simulink model "mech_interface_crate_trans"  (R2015a)
settings: Solver=ode15s  StartTime=0.0  StopTime=10.0  RelTol=1e-3
PostLoadFcn:
  | mech_crate_transfer_param
model workspace (MAT data in the model file):
  A_a = 0.05
  A_b = 0.5
  A_c = 0.05
  M_a = 1
  I_a = [0.0841666666667  0  0; 0  0.00166666666667  0; 0  0  0.0841666666667]
  C_a = 0.25
  C_b = 0.05
  C_c = 0.05
  M_c = 5
  I_c = [0.00833333333333  0  0; 0  0.108333333333  0; 0  0  0.108333333333]
undefined symbols (not defined in the file): sigbuilder_block
libraries: mblibv1 x17, fl_lib x10, nesl_utility x4
Description:
  | Hydraulically Operated Crate Transfer Mechanism
  | 
  | This example shows a hydraulically operated four bar linkage that transfers crates between platforms of different heights. The Body Force Interface subsystem uses a Prismatic-Translational Interface block with Spherical and Prismatic joints to connect a hydraulic cylinder between Ground C and Body B.
  | 
  | The hydraulic circuit is modeled in Simscape(TM). The rest of the mechanism is modeled in SimMechanics(TM).
  | 
  | Copyright 2008-2014 The MathWorks, Inc.
settings Model: CovSFcnEnable=off  Creator=MathWorks  LastModifiedBy=psanghvi
settings SolverCC: MaxOrder=3  SolverResetMethod=Robust
settings DataIOCC: SignalLoggingSaveFormat=ModelDataLogs  OutputOption=SpecifiedOutputTimes  OutputTimes=[0:0.05:10]
settings OptimizationCC: ExpressionDepthLimit=2147483647  InitFltsAndDblsToZero=on
settings DebuggingCC: AlgebraicLoopMsg=none  UnderspecifiedInitializationDetection=Classic  MergeDetectMultiDrivingBlocksExec=none  FcnCallInpInsideContextMsg=UseLocalSettings  StateNameClashWarn=warning
settings GRTTargetCC: TargetFcnLib=ansi_tfl_tmw_new.mat  CombineOutputUpdateFcns=off  GRTInterface=on
settings SimMechanicsCC: WarnOnRedundantConstraints=off  VisOnUpdateDiagram=on  VisDuringSimulation=on  AnimationDelay=0  LastVizWinPosition=[680 677 559 420]  CamPosition=[0.138538;0.4511;12.0268;]  CamTarget=[0.138538;0.4511;0;]  CamUpVector=[0;1;0;]  CamHeight=1.87351  VisBackgroundColor=[0.9;0.9;0.95;]  DefaultBodyColor=[1;0;0;]  OVRRIDBodyVisualizationType=CONVHULL

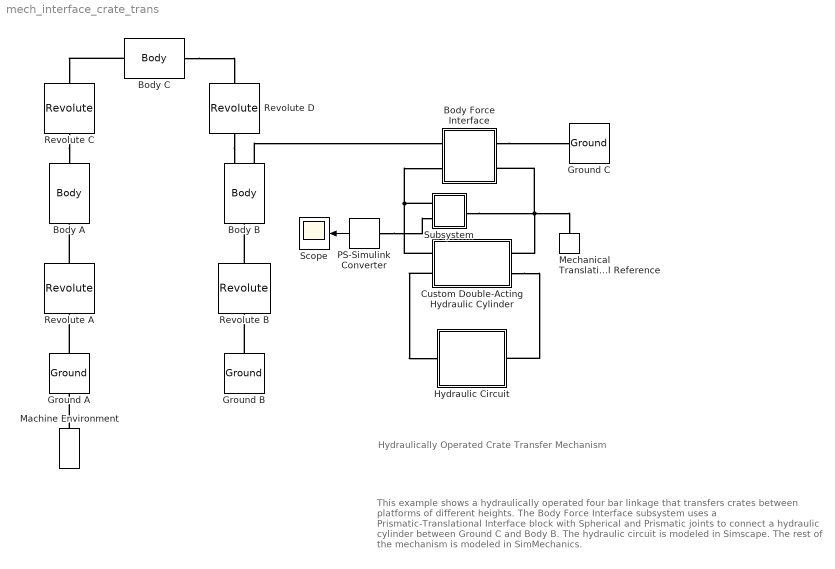
== system mech_interface_crate_trans ==
  note: Hydraulically Operated Crate Transfer Mechanism
  note: This example shows a hydraulically operated four bar linkage that
      | transfers crates between platforms of different heights. The Body Force Interface
      | subsystem uses a Prismatic-Translational Interface block with Spherical and Prismatic
      | joints to connect a hydraulic cylinder between Ground C and Body B.
      |
      | The hydraulic circuit is modeled in Simscape.
      | The rest of the mechanism is modeled in SimMechanics.
  Body A : mblibv1/Bodies/Body  LConnTagsString=CS1  RConnTagsString=CS2  UpdateFromCAD=off  DialogClass=MechanicalBodyBlock  Mass=M_a  MassUnits=kg  InertiaUnits=kg*m^2  Inertia=I_a  Shape=Cylinder  ShapeDims=[1 1]  ShapeUnits=m  ShapeUse=false  Density=1  DensityUnits=kg/m^3  DensityUse=false  GraphicsMode=MACHINE_DEFAULT  BodyColorSelMode=MACHINE_DEFAULT  BodyColor=[1 0 0]  AttachedToCS=CG  CG=Left$CG$[0 A_b 0]$CS1$CS1$m$[0 0 0]$Euler X-Y-Z$deg$WORLD$false  WorkingFrames=Left$CS1$[0.0 0 0]$Adjoining$Adjoining$m$[0 0 0]$Euler X-Y-Z$deg$WORLD$true#Right$CS2$[0 2*A_b 0]$CS1$CS1$m$[0 0 0]$Euler X-Y-Z$deg$WORLD$true  CGPos=[0 A_b 0]  CGRot=[0 0 0]  CS0Pos=[]  CS0Rot=[]  CS1Pos=[0.0 0 0]  CS1Rot=[0 0 0]  CS2Pos=[0 2*A_b 0]  CS2Rot=[0 0 0]  CS3Pos=[]  CS3Rot=[]  CS4Pos=[]  CS4Rot=[]  CS5Pos=[]  CS5Rot=[]  CS6Pos=[]  CS6Rot=[]  CS7Pos=[]  CS7Rot=[]  CS8Pos=[]  CS8Rot=[]  CS9Pos=[]  CS9Rot=[]  CS10Pos=[]  CS10Rot=[]  CS11Pos=[]  CS11Rot=[]  CS12Pos=[]  CS12Rot=[]  CS13Pos=[]  CS13Rot=[]  CS14Pos=[]  CS14Rot=[]  CS15Pos=[]  CS15Rot=[]  CS16Pos=[]  CS16Rot=[]  CS17Pos=[]  CS17Rot=[]  CS18Pos=[]  CS18Rot=[]  CS19Pos=[]  CS19Rot=[]  CS20Pos=[]  CS20Rot=[]
  Body B : mblibv1/Bodies/Body  LConnTagsString=CS1  RConnTagsString=CS2|CS3  UpdateFromCAD=off  DialogClass=MechanicalBodyBlock  Mass=M_a  MassUnits=kg  InertiaUnits=kg*m^2  Inertia=I_a  Shape=Cylinder  ShapeDims=[1 1]  ShapeUnits=m  ShapeUse=false  Density=1  DensityUnits=kg/m^3  DensityUse=false  GraphicsMode=MACHINE_DEFAULT  BodyColorSelMode=MACHINE_DEFAULT  BodyColor=[1 0 0]  AttachedToCS=CG  CG=Left$CG$[0 A_b 0]$CS1$CS1$m$[0 0 0]$Euler X-Y-Z$deg$WORLD$false  WorkingFrames=Left$CS1$[0 0 0]$Adjoining$Adjoining$m$[0 0 0]$Euler X-Y-Z$deg$WORLD$true#Right$CS2$[0 2*A_b 0]$CS1$CS1$m$[0 0 0]$Euler X-Y-Z$deg$WORLD$true#Right$CS3$[0 0 0]$CG$CG$m$[0 0 0]$Euler X-Y-Z$deg$WORLD$true  CGPos=[0 A_b 0]  CGRot=[0 0 0]  CS0Pos=[]  CS0Rot=[]  CS1Pos=[0 0 0]  CS1Rot=[0 0 0]  CS2Pos=[0 2*A_b 0]  CS2Rot=[0 0 0]  CS3Pos=[0 0 0]  CS3Rot=[0 0 0]  CS4Pos=[]  CS4Rot=[]  CS5Pos=[]  CS5Rot=[]  CS6Pos=[]  CS6Rot=[]  CS7Pos=[]  CS7Rot=[]  CS8Pos=[]  CS8Rot=[]  CS9Pos=[]  CS9Rot=[]  CS10Pos=[]  CS10Rot=[]  CS11Pos=[]  CS11Rot=[]  CS12Pos=[]  CS12Rot=[]  CS13Pos=[]  CS13Rot=[]  CS14Pos=[]  CS14Rot=[]  CS15Pos=[]  CS15Rot=[]  CS16Pos=[]  CS16Rot=[]  CS17Pos=[]  CS17Rot=[]  CS18Pos=[]  CS18Rot=[]  CS19Pos=[]  CS19Rot=[]  CS20Pos=[]  CS20Rot=[]
  Body C : mblibv1/Bodies/Body  LConnTagsString=CS1  RConnTagsString=CS2  UpdateFromCAD=off  DialogClass=MechanicalBodyBlock  Mass=M_c  MassUnits=kg  InertiaUnits=kg*m^2  Inertia=I_c  Shape=Cylinder  ShapeDims=[1 1]  ShapeUnits=m  ShapeUse=false  Density=1  DensityUnits=kg/m^3  DensityUse=false  GraphicsMode=MACHINE_DEFAULT  BodyColorSelMode=MACHINE_DEFAULT  BodyColor=[1 0 0]  AttachedToCS=CG  CG=Left$CG$[C_a 0 0]$CS1$CS1$m$[0 0 0]$Euler X-Y-Z$deg$WORLD$false  WorkingFrames=Left$CS1$[0.0 0 0]$Adjoining$Adjoining$m$[0 0 0]$Euler X-Y-Z$deg$WORLD$true#Right$CS2$[2*C_a 0 0]$CS1$CS1$m$[0 0 0]$Euler X-Y-Z$deg$WORLD$true  CGPos=[C_a 0 0]  CGRot=[0 0 0]  CS0Pos=[]  CS0Rot=[]  CS1Pos=[0.0 0 0]  CS1Rot=[0 0 0]  CS2Pos=[2*C_a 0 0]  CS2Rot=[0 0 0]  CS3Pos=[]  CS3Rot=[]  CS4Pos=[]  CS4Rot=[]  CS5Pos=[]  CS5Rot=[]  CS6Pos=[]  CS6Rot=[]  CS7Pos=[]  CS7Rot=[]  CS8Pos=[]  CS8Rot=[]  CS9Pos=[]  CS9Rot=[]  CS10Pos=[]  CS10Rot=[]  CS11Pos=[]  CS11Rot=[]  CS12Pos=[]  CS12Rot=[]  CS13Pos=[]  CS13Rot=[]  CS14Pos=[]  CS14Rot=[]  CS15Pos=[]  CS15Rot=[]  CS16Pos=[]  CS16Rot=[]  CS17Pos=[]  CS17Rot=[]  CS18Pos=[]  CS18Rot=[]  CS19Pos=[]  CS19Rot=[]  CS20Pos=[]  CS20Rot=[]
  Body Force Interface : Subsystem
  Custom Double-Acting Hydraulic Cylinder : Subsystem  mask(Hydraulic Double-Acting Cylinder, Custom Model){area_A=0.001, area_B=5e-4, stroke=1, init_pos=0.5, stiffness=1e6, damping=150}
      mask prompts: area_A "Area A (m^2)"; area_B "Area B (m^2)"; stroke "Stroke (m)"; init_pos "Initial position (m)"; stiffness "Contact stiffness (N/m)"; damping "Contact damping (N*s/m)"
      mask help: The model is built entirely of Foundation Library blocks and accounts for hard stops and fluid consumption due to piston motion.
      mask Display:
      | plot([127.790967235342;156.136468285695;156.136468285695;127.790967235342;127.790967235342], [113.618216710165;113.618216710165;56.927214609459;56.927214609459;113.618216710165])
      | plot([227.000220911577;227.000220911577;56.927214609459;56.927214609459;227.000220911577;227.000220911577], [99.4454661849886;113.618216710165;113.618216710165;56.927214609459;56.927214609459;71.0999651346356])
      | plot([156.136468285695;297.86397353746;297.86397353746;156.136468285695;156.136468285695], [99.4454661849886;99.4454661849886;71.0999651346356;71.0999651346356;99.4454661849886])
      | plot([56.927214609459;28.581713559106;56.927214609459], [113.618216710165;85.2727156598121;56.927214609459])
      | plot([28.581713559106;0.236212508752942], [85.2727156598121;85.2727156598121])
      | plot([297.86397353746;326.209474587813], [85.2727156598121;85.2727156598121])
      | plot([0.236212508752942;71.0999651346356;71.0999651346356], [28.581713559106;28.581713559106;56.927214609459])
      | plot([212.827470386401;212.827470386401;323.374924482778], [56.927214609459;28.581713559106;28.581713559106])
      | patch([0;326.445687096566;326.445687096566;0;0;0.472425017505884;0.472425017505884;325.97326207906;325.97326207906;0.472425017505884;0], [113.854429218918;113.854429218918;0;0;113.854429218918;113.382004201412;0.472425017505884;0.472425017505884;113.382004201412;113.382004201412;113.854429218918], [1;1;1])
      | ;
  Ground A : mblibv1/Bodies/Ground  UpdateFromCAD=off  LeftPortType=env  RightPortType=workingframe  PhysicalDomain=Mechanical  DialogClass=GroundBlock  CoordPosition=[0 0 0]  CoordPositionUnits=m  StateVectorMgrId=-1  MachineId=[0 0]  ShowEnvPort=on  ParameterChecksum=[2928839484, 1749172837, 1649258051, 964539551]  TopologyChecksum=[4150982369, 548530894, 407794712, 2107293366]
  Ground B : mblibv1/Bodies/Ground  UpdateFromCAD=off  LeftPortType=env  RightPortType=workingframe  PhysicalDomain=Mechanical  DialogClass=GroundBlock  CoordPosition=[0.5 0 0]  CoordPositionUnits=m  StateVectorMgrId=-1  MachineId=[0 0]  ShowEnvPort=off  ParameterChecksum=[0 0 0 0]  TopologyChecksum=[0 0 0 0]
  Ground C : mblibv1/Bodies/Ground  UpdateFromCAD=off  LeftPortType=env  RightPortType=workingframe  PhysicalDomain=Mechanical  DialogClass=GroundBlock  CoordPosition=[1 1 0]  CoordPositionUnits=m  StateVectorMgrId=-1  MachineId=[0 0]  ShowEnvPort=off  ParameterChecksum=[0 0 0 0]  TopologyChecksum=[0 0 0 0]
  Hydraulic Circuit : Subsystem
  Machine Environment : mblibv1/Bodies/Machine Environment  Tag=Factory ground  PortType=env  PhysicalDomain=Mechanical  DialogTemplateClass=MECH.MachineEnvironment  SyncWhenCopied=off  Gravity=[0 0 0]  GravityUnits=m/s^2  GravityAsSignal=off  Dimensionality=Auto-detect  AnalysisType=Forward dynamics  LinearAssemblyTolerance=1e-3  LinearAssemblyToleranceUnits=m  AngularAssemblyTolerance=1e-3  AngularAssemblyToleranceUnits=rad  ConstraintSolverType=Stabilizing  ConstraintRelTolerance=1e-4  ConstraintAbsTolerance=1e-4  UseRobustSingularityHandling=off  RedundancyAnalysisToleranceType=Automatically select tolerance  RedundancyAnalysisTolerance=1e-14  StatePerturbationType=Fixed  PerturbationSize=1e-5  VisualizeMachine=on  BodyVisualizationType=Use model default body geometries  BodyColorSelMode=Use model default  DefaultBodyColor=[1 0 0]
  Mechanical Translational Reference : fl_lib/Mechanical/Translational Elements/Mechanical Translational Reference
  PS-Simulink Converter : nesl_utility/PS-Simulink Converter  PhysicalDomain=network_engine_domain  SubClassName=ps_output  LeftPortType=input  RightPortType=output  PseudoPeriodic=off  Frequencies=[]  Unit=1  AffineConversion=off
  Revolute A : mblibv1/Joints/Revolute  LConnTagsString=__newl0  RConnTagsString=__newr0  UpdateFromCAD=off  NumSAPorts=0  CutJoint=off  MarkAsCut=off  Primitives=prismatic  PrimitiveProps=R1$World$[0 0 1]$revolute  DialogClass=JointBlock  R1Axis=[0 0 1]
  Revolute B : mblibv1/Joints/Revolute  LConnTagsString=__newl0  RConnTagsString=__newr0  UpdateFromCAD=off  NumSAPorts=0  CutJoint=off  MarkAsCut=off  Primitives=prismatic  PrimitiveProps=R1$World$[0 0 1]$revolute  DialogClass=JointBlock  R1Axis=[0 0 1]
  Revolute C : mblibv1/Joints/Revolute  LConnTagsString=__newl0  RConnTagsString=__newr0  UpdateFromCAD=off  NumSAPorts=0  CutJoint=off  MarkAsCut=off  Primitives=prismatic  PrimitiveProps=R1$WORLD$[0 0 1]$revolute  DialogClass=JointBlock  R1Axis=[0 0 1]
  Revolute D : mblibv1/Joints/Revolute  LConnTagsString=__newl0  RConnTagsString=__newr0  UpdateFromCAD=off  NumSAPorts=0  CutJoint=off  MarkAsCut=off  Primitives=prismatic  PrimitiveProps=R1$World$[0 0 1]$revolute  DialogClass=JointBlock  R1Axis=[0 0 1]
  Scope : Scope
      settings: TimeRange=10  YMin=-0.05  YMax=0.15
  Subsystem : Subsystem
  wires:
  PS-Simulink Converter/1 -> Scope/1
  connections:
  Ground A/RConn1 -- Revolute A/LConn1
  Revolute A/RConn1 -- Body A/LConn1
  Revolute B/RConn1 -- Body B/LConn1
  Ground B/RConn1 -- Revolute B/LConn1
  Revolute C/LConn1 -- Body A/RConn1
  Body C/LConn1 -- Revolute C/RConn1
  Revolute D/LConn1 -- Body B/RConn1
  Body C/RConn1 -- Revolute D/RConn1
  Body B/RConn2 -- Body Force Interface/LConn1
  Machine Environment/RConn1 -- Ground A/LConn1
  Custom Double-Acting Hydraulic Cylinder/RConn2 -- Hydraulic Circuit/LConn1
  Custom Double-Acting Hydraulic Cylinder/LConn2 -- Hydraulic Circuit/RConn1
  Custom Double-Acting Hydraulic Cylinder/LConn1 -- Body Force Interface/RConn2 -- Subsystem/RConn1 -- Mechanical Translational Reference/LConn1
  Custom Double-Acting Hydraulic Cylinder/RConn1 -- Subsystem/LConn1 -- Body Force Interface/LConn2
  Body Force Interface/RConn1 -- Ground C/RConn1
  PS-Simulink Converter/LConn1 -- Subsystem/LConn2

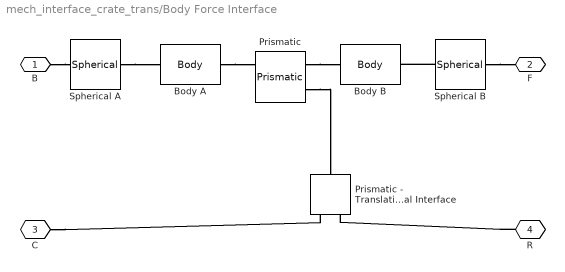
== system mech_interface_crate_trans/Body Force Interface ==
  Body A : mblibv1/Bodies/Body  LConnTagsString=CS1  RConnTagsString=CS2  UpdateFromCAD=off  DialogClass=MechanicalBodyBlock  Mass=0.1  MassUnits=kg  InertiaUnits=kg*m^2  Inertia=1e-3*[0.1 0 0;0 3 0; 0 0 3]  Shape=Cylinder  ShapeDims=[1 1]  ShapeUnits=m  ShapeUse=false  Density=1  DensityUnits=kg/m^3  DensityUse=false  GraphicsMode=MACHINE_DEFAULT  BodyColorSelMode=MACHINE_DEFAULT  BodyColor=[1 0 0]  AttachedToCS=CG  CG=Left$CG$[sqrt(2)*0.5/2 0 0]$CS1$CS1$m$[0 0 0]$Euler X-Y-Z$deg$CS1$false$none  WorkingFrames=Left$CS1$[0 0 0]$Adjoining$Adjoining$m$[0 0 45]$Euler X-Y-Z$deg$WORLD$true$none#Right$CS2$[sqrt(2)*0.5 0 0]$CS1$CS1$m$[0 0 0]$Euler X-Y-Z$deg$CS1$true$none  CGPos=[sqrt(2)*0.5/2 0 0]  CGRot=[0 0 0]  CS0Pos=[]  CS0Rot=[]  CS1Pos=[0 0 0]  CS1Rot=[0 0 45]  CS2Pos=[sqrt(2)*0.5 0 0]  CS2Rot=[0 0 0]  CS3Pos=[]  CS3Rot=[]  CS4Pos=[]  CS4Rot=[]  CS5Pos=[]  CS5Rot=[]  CS6Pos=[]  CS6Rot=[]  CS7Pos=[]  CS7Rot=[]  CS8Pos=[]  CS8Rot=[]  CS9Pos=[]  CS9Rot=[]  CS10Pos=[]  CS10Rot=[]  CS11Pos=[]  CS11Rot=[]  CS12Pos=[]  CS12Rot=[]  CS13Pos=[]  CS13Rot=[]  CS14Pos=[]  CS14Rot=[]  CS15Pos=[]  CS15Rot=[]  CS16Pos=[]  CS16Rot=[]  CS17Pos=[]  CS17Rot=[]  CS18Pos=[]  CS18Rot=[]  CS19Pos=[]  CS19Rot=[]  CS20Pos=[]  CS20Rot=[]
  Body B : mblibv1/Bodies/Body  LConnTagsString=CS1  RConnTagsString=CS2  UpdateFromCAD=off  DialogClass=MechanicalBodyBlock  Mass=0.1  MassUnits=kg  InertiaUnits=kg*m^2  Inertia=1e-3*[0.1 0 0;0 3 0; 0 0 3]  Shape=Cylinder  ShapeDims=[1 1]  ShapeUnits=m  ShapeUse=false  Density=1  DensityUnits=kg/m^3  DensityUse=false  GraphicsMode=MACHINE_DEFAULT  BodyColorSelMode=MACHINE_DEFAULT  BodyColor=[1 0 0]  AttachedToCS=CG  CG=Left$CG$[sqrt(2)*0.5/2 0 0]$CS1$CS1$m$[0 0 0]$Euler X-Y-Z$deg$CS1$false$none  WorkingFrames=Left$CS1$[-sqrt(2)*0.5 0 0]$Adjoining$Adjoining$m$[0 0 0]$Euler X-Y-Z$deg$Adjoining$true$none#Right$CS2$[sqrt(2)*0.5 0 0]$CS1$CS1$m$[0 0 0]$Euler X-Y-Z$deg$CS1$true$none  CGPos=[sqrt(2)*0.5/2 0 0]  CGRot=[0 0 0]  CS0Pos=[]  CS0Rot=[]  CS1Pos=[-sqrt(2)*0.5 0 0]  CS1Rot=[0 0 0]  CS2Pos=[sqrt(2)*0.5 0 0]  CS2Rot=[0 0 0]  CS3Pos=[]  CS3Rot=[]  CS4Pos=[]  CS4Rot=[]  CS5Pos=[]  CS5Rot=[]  CS6Pos=[]  CS6Rot=[]  CS7Pos=[]  CS7Rot=[]  CS8Pos=[]  CS8Rot=[]  CS9Pos=[]  CS9Rot=[]  CS10Pos=[]  CS10Rot=[]  CS11Pos=[]  CS11Rot=[]  CS12Pos=[]  CS12Rot=[]  CS13Pos=[]  CS13Rot=[]  CS14Pos=[]  CS14Rot=[]  CS15Pos=[]  CS15Rot=[]  CS16Pos=[]  CS16Rot=[]  CS17Pos=[]  CS17Rot=[]  CS18Pos=[]  CS18Rot=[]  CS19Pos=[]  CS19Rot=[]  CS20Pos=[]  CS20Rot=[]
  Prismatic : mblibv1/Joints/Prismatic  LConnTagsString=__newl0|SA1  RConnTagsString=__newr0|SA1  UpdateFromCAD=off  NumSAPorts=2  CutJoint=off  MarkAsCut=off  Primitives=prismatic  PrimitiveProps=P1$Base$[1 0 0]$prismatic  DialogClass=JointBlock  P1Axis=[1 0 0]
  Prismatic - Translational Interface : mblibv1/Interface  Elements/Prismatic - Translational Interface  UpdateFromCAD=off  DialogClass=PrismaticTranslationalInterface  Primitive=P1  InputFiltering=off  SimscapeFilterOrder=1  InputFilterTimeConstant=0.001
  "Spherical A " : mblibv1/Joints/Spherical  LConnTagsString=__newl0  RConnTagsString=__newr0  UpdateFromCAD=off  NumSAPorts=0  CutJoint=off  MarkAsCut=off  Primitives=spherical  PrimitiveProps=S$WORLD$[0 0 0]$spherical  DialogClass=JointBlock  SAxis=[0 0 0]
  Spherical B : mblibv1/Joints/Spherical  LConnTagsString=__newl0  RConnTagsString=__newr0  UpdateFromCAD=off  NumSAPorts=0  CutJoint=off  MarkAsCut=off  Primitives=spherical  PrimitiveProps=S$World$[0 0 0]$spherical  DialogClass=JointBlock  SAxis=[0 0 0]
  B : PMIOPort  Port=1  Side=Left
  F : PMIOPort  Port=2  Side=Right
  C : PMIOPort  Port=3  Side=Left
  R : PMIOPort  Port=4  Side=Right
  connections:
  R/RConn1 -- Prismatic - Translational Interface/LConn2
  C/RConn1 -- Prismatic - Translational Interface/LConn1
  B/RConn1 -- "Spherical A "/LConn1
  "Spherical A "/RConn1 -- Body A/LConn1
  Body A/RConn1 -- Prismatic/RConn1
  Prismatic/LConn1 -- Body B/LConn1
  Prismatic/LConn2 -- Prismatic - Translational Interface/RConn1
  Spherical B/RConn1 -- F/RConn1
  Spherical B/LConn1 -- Body B/RConn1

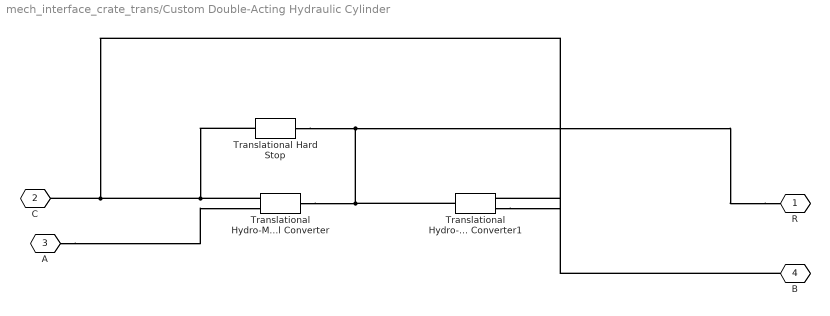
== system mech_interface_crate_trans/Custom Double-Acting Hydraulic Cylinder ==
  Translational Hydro-Mechanical Converter : fl_lib/Hydraulic/Hydraulic Elements/Translational Hydro-Mechanical Converter  area=area_A m^2  or=1  compressibility=0  init_pos=0 m  V_dead=1e-4 m^3  k_sh=1.4  initial_pressure=0 Pa
  Translational Hydro-Mechanical Converter1 : fl_lib/Hydraulic/Hydraulic Elements/Translational Hydro-Mechanical Converter  area=area_B m^2  or=2  compressibility=0  init_pos=0 m  V_dead=1e-4 m^3  k_sh=1.4  initial_pressure=0 Pa
  Translational Hard Stop : fl_lib/Mechanical/Translational Elements/Translational Hard Stop  upper_bnd=stroke - init_pos m  lower_bnd=-init_pos m  stiff_up=stiffness N/m  stiff_low=stiffness N/m  D_up=damping N/(m/s)  D_low=damping N/(m/s)  v_specify=off  v_priority=High  v=0 m/s  f_specify=off  f_priority=High  f=0 N  x_specify=on  x_priority=High  x=0 m
  R : PMIOPort  Tag=PMCPort  Port=1  Side=Right
  C : PMIOPort  Tag=PMCPort  Port=2  Side=Left
  A : PMIOPort  Tag=PMCPort  Port=3  Side=Left
  B : PMIOPort  Tag=PMCPort  Port=4  Side=Right
  connections:
  R/RConn1 -- Translational Hydro-Mechanical Converter1/RConn1 -- Translational Hydro-Mechanical Converter/RConn1 -- Translational Hard Stop/LConn1
  Translational Hydro-Mechanical Converter1/LConn1 -- Translational Hard Stop/RConn1 -- Translational Hydro-Mechanical Converter/LConn1 -- C/RConn1
  A/RConn1 -- Translational Hydro-Mechanical Converter/LConn2
  B/RConn1 -- Translational Hydro-Mechanical Converter1/LConn2

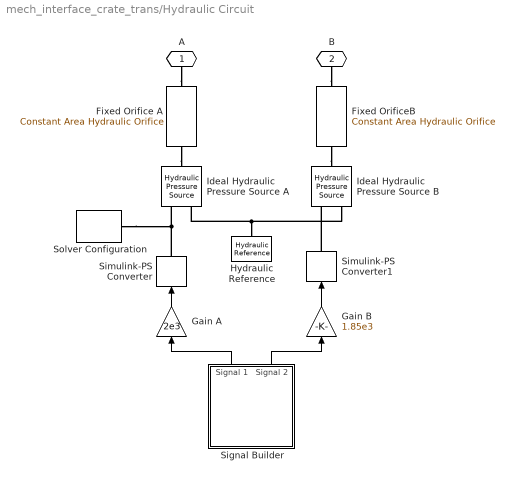
== system mech_interface_crate_trans/Hydraulic Circuit ==
  Fixed Orifice A : fl_lib/Hydraulic/Hydraulic Elements/Constant Area Hydraulic Orifice  area=1e-04 m^2  C_d=0.7  Re_cr=12  D_h=0.0113 m  p_cr=1 Pa  q_specify=off  q_priority=High  q=1 m^3/s  p_specify=off  p_priority=High  p=0 Pa
  Fixed OrificeB : fl_lib/Hydraulic/Hydraulic Elements/Constant Area Hydraulic Orifice  area=1e-04 m^2  C_d=0.7  Re_cr=12  D_h=0.0113 m  p_cr=1 Pa  q_specify=off  q_priority=High  q=1 m^3/s  p_specify=off  p_priority=High  p=0 Pa
  Gain A : Gain  Gain=2e3
  Gain B : Gain  Gain=1.85e3
  Hydraulic Reference : fl_lib/Hydraulic/Hydraulic Elements/Hydraulic Reference
  Ideal Hydraulic Pressure Source A : fl_lib/Hydraulic/Hydraulic Sources/Hydraulic Pressure Source
  Ideal Hydraulic Pressure Source B : fl_lib/Hydraulic/Hydraulic Sources/Hydraulic Pressure Source
  Signal Builder : Subsystem  Tag=STV Subsys  LoadFcn=sigbuilder_block('load');  StartFcn=sigbuilder_block('start');  StopFcn=sigbuilder_block('stop');  ClipboardFcn=sigbuilder_block('clipboard');  mask(Sigbuilder block){}
      mask help: Sigbuilder GUI
      mask init:
      | if ~strcmp(get_param(bdroot(gcbh),'SimulationStatus'),'stopped') tuvar = sigbuilder_block('maskInit'); end
      settings: CopyFcn=sigbuilder_block('copy');  DeleteFcn=sigbuilder_block('delete');  ModelCloseFcn=sigbuilder_block('modelClose');  PreSaveFcn=sigbuilder_block('preSave');  PauseFcn=sigbuilder_block('pause')  ContinueFcn=sigbuilder_block('continue')  NameChangeFcn=sigbuilder_block('namechange');  OpenFcn=sigbuilder_block('open',[388.5 359.25 550.5 371.25 ]);  CloseFcn=sigbuilder_block('close');
      mask Display: plot(0,0,100,100,[10,10,40,40,10],[80,20,20,80,80],[40,10],[50,50], [40,27,10],[65,72,56],[40,25,25,10],[28,28,43,43]);
  Simulink-PS Converter : nesl_utility/Simulink-PS Converter  PhysicalDomain=network_engine_domain  SubClassName=ps_input  LeftPortType=input  RightPortType=output  PseudoPeriodic=off  Frequencies=[]  NoiseDistribution=none  NoiseParameters=[]  Unit=N/m^2  AffineConversion=off  InputFiltering=off  SimscapeFilterOrder=1  InputFilterTimeConstant=.001  UdotUserProvided=0
  Simulink-PS Converter1 : nesl_utility/Simulink-PS Converter  PhysicalDomain=network_engine_domain  SubClassName=ps_input  LeftPortType=input  RightPortType=output  PseudoPeriodic=off  Frequencies=[]  NoiseDistribution=none  NoiseParameters=[]  Unit=N/m^2  AffineConversion=off  InputFiltering=off  SimscapeFilterOrder=1  InputFilterTimeConstant=.001  UdotUserProvided=0
  Solver Configuration : nesl_utility/Solver Configuration  PhysicalDomain=network_engine_domain  SubClassName=solver  LeftPortType=input  RightPortType=generic  Accelerate=off  Tones=[]  Harmonics=[]  SimulateNoise=off  Profile=off  UseLocalSampling=off  EnableSwitchedLinearOptims=on  FrequencyDomain=off  UseCCode=off  RelTol=0.001  AbsTol=1e-06  MinStep=1e-09  ToWorkspace=off  RevertToSquareIcSolve=off  NumHomotopyIterations=100  DoDC=off  ResidualTolerance=1e-9  UseLocalSolver=off  LocalSolverChoice=NE_BACKWARD_EULER_ADVANCER  LocalSolverSampleTime=.001  DoFixedCost=off  MaxNonlinIter=12  MaxModeIter=2  LinearAlgebra=Sparse  DelaysMemoryBudget=1024  AutomaticFiltering=on  FilteringTimeConstant=0.001
  A : PMIOPort  Port=1  Side=Right
  B : PMIOPort  Port=2  Side=Left
  wires:
  Signal Builder/2(Signal 2) -> Gain B/1
  Signal Builder/1(Signal 1) -> Gain A/1
  Gain A/1 -> Simulink-PS Converter/1
  Gain B/1 -> Simulink-PS Converter1/1
  connections:
  Fixed OrificeB/RConn1 -- Ideal Hydraulic Pressure Source B/LConn1
  Simulink-PS Converter/RConn1 -- Ideal Hydraulic Pressure Source A/RConn1 -- Solver Configuration/RConn1
  Simulink-PS Converter1/RConn1 -- Ideal Hydraulic Pressure Source B/RConn1
  A/RConn1 -- Fixed Orifice A/RConn1
  B/RConn1 -- Fixed OrificeB/LConn1
  Fixed Orifice A/LConn1 -- Ideal Hydraulic Pressure Source A/LConn1
  Ideal Hydraulic Pressure Source B/RConn2 -- Ideal Hydraulic Pressure Source A/RConn2 -- Hydraulic Reference/LConn1

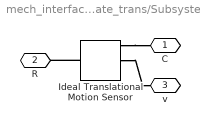
== system mech_interface_crate_trans/Subsystem ==
  Ideal Translational Motion Sensor : fl_lib/Mechanical/Mechanical Sensors/Ideal Translational Motion Sensor  offset=0 m
  C : PMIOPort  Port=1  Side=Right
  R : PMIOPort  Port=2  Side=Left
  v : PMIOPort  Port=3  Side=Left
  connections:
  Ideal Translational Motion Sensor/LConn1 -- R/RConn1
  Ideal Translational Motion Sensor/RConn1 -- C/RConn1
  Ideal Translational Motion Sensor/RConn2 -- v/RConn1

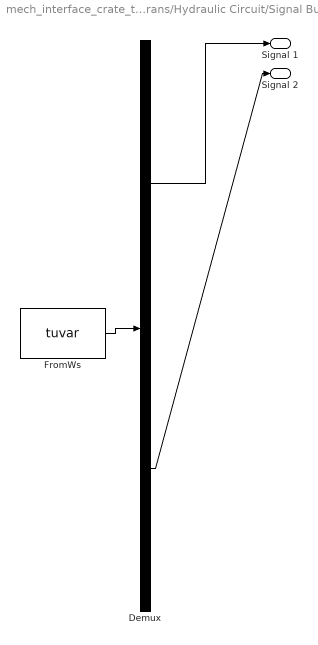
== system mech_interface_crate_trans/Hydraulic Circuit/Signal Builder ==
  Demux : Demux  Tag=STV Demux  Outputs=2
  FromWs : FromWorkspace  Tag=STV FromWs  VariableName=tuvar  SampleTime=0
      SigBuilderData=|
      | common.afterFinalStr = 'Extrapolate'
      | common.sampleTime = 0
      | dataSet.timeRange = [0 10]
      | dataSet.name = 'Group 1'
      | sbobj.Groups.Name = 'Group 1'
      | sbobj.Groups.Signals(1).Name = 'Signal 1'
      | sbobj.Groups.Signals(1).XData = [0 1.02 1.02 2 3 4 5.02 10]
      | sbobj.Groups.Signals(1).YData = [0 0 0.01 0.79 1 0.79 0.01 0]
      | sbobj.Groups.Signals(2).Name = 'Signal 2'
      | sbobj.Groups.Signals(2).XData = [0 4 5 5.98 6.98 7.98 10]
      | sbobj.Groups.Signals(2).YData = [0 0 0.79 0.997010505051 0.78 0 0]
  Signal 1 : Outport  Tag=STV Outport
  Signal 2 : Outport  Tag=STV Outport  Port=2
  wires:
  Demux/1 -> Signal 1/1
  FromWs/1 -> Demux/1
  Demux/2 -> Signal 2/1
